simulink model "sampleModel7424_pp_1_1"  (R2018a)
settings: Solver=VariableStepAuto  StartTime=0.0  StopTime=10.0  RelTol=1e-3
undefined symbols (not defined in the file): DiscIntNeverNeededParam
libraries: simulink x211
(part 7 of 7)

== matlab function sampleModel7424_pp_1_1/emi_267 ==
  data: o input; e input
function  fcn(o, e)
o_inv = o^-1;
e_inv = e^-1;

emsg = 'sampleModel7424_pp_1_1/emi_267';
 
if(o == e)
    assert(o_inv == e_inv, [emsg ' ; o_inv~=e_inv']);
    return;
end
 
if(o_inv > 0)
    assert(e_inv < 0, [emsg ' ; e_inv>=0']);
else
    assert(e_inv > 0, [emsg ' ; e_inv<=0']);
end

== matlab function sampleModel7424_pp_1_1/cfblk148/cfblk19/emi_269 ==
  data: o input; e input
function  fcn(o, e)
o_inv = o^-1;
e_inv = e^-1;

emsg = 'sampleModel7424_pp_1_1/cfblk148/cfblk19/emi_269';
 
if(o == e)
    assert(o_inv == e_inv, [emsg ' ; o_inv~=e_inv']);
    return;
end
 
if(o_inv > 0)
    assert(e_inv < 0, [emsg ' ; e_inv>=0']);
else
    assert(e_inv > 0, [emsg ' ; e_inv<=0']);
end

== matlab function sampleModel7424_pp_1_1/cfblk140/emi_271 ==
  data: o input; e input
function  fcn(o, e)
o_inv = o^-1;
e_inv = e^-1;

emsg = 'sampleModel7424_pp_1_1/cfblk140/emi_271';
 
if(o == e)
    assert(o_inv == e_inv, [emsg ' ; o_inv~=e_inv']);
    return;
end
 
if(o_inv > 0)
    assert(e_inv < 0, [emsg ' ; e_inv>=0']);
else
    assert(e_inv > 0, [emsg ' ; e_inv<=0']);
end

== matlab function sampleModel7424_pp_1_1/emi_273 ==
  data: o input; e input
function  fcn(o, e)
o_inv = o^-1;
e_inv = e^-1;

emsg = 'sampleModel7424_pp_1_1/emi_273';
 
if(o == e)
    assert(o_inv == e_inv, [emsg ' ; o_inv~=e_inv']);
    return;
end
 
if(o_inv > 0)
    assert(e_inv < 0, [emsg ' ; e_inv>=0']);
else
    assert(e_inv > 0, [emsg ' ; e_inv<=0']);
end

== matlab function sampleModel7424_pp_1_1/cfblk124/emi_275 ==
  data: o input; e input
function  fcn(o, e)
o_inv = o^-1;
e_inv = e^-1;

emsg = 'sampleModel7424_pp_1_1/cfblk124/emi_275';
 
if(o == e)
    assert(o_inv == e_inv, [emsg ' ; o_inv~=e_inv']);
    return;
end
 
if(o_inv > 0)
    assert(e_inv < 0, [emsg ' ; e_inv>=0']);
else
    assert(e_inv > 0, [emsg ' ; e_inv<=0']);
end

== matlab function sampleModel7424_pp_1_1/cfblk134/cfblk19/emi_277 ==
  data: o input; e input
function  fcn(o, e)
o_inv = o^-1;
e_inv = e^-1;

emsg = 'sampleModel7424_pp_1_1/cfblk134/cfblk19/emi_277';
 
if(o == e)
    assert(o_inv == e_inv, [emsg ' ; o_inv~=e_inv']);
    return;
end
 
if(o_inv > 0)
    assert(e_inv < 0, [emsg ' ; e_inv>=0']);
else
    assert(e_inv > 0, [emsg ' ; e_inv<=0']);
end

== matlab function sampleModel7424_pp_1_1/cfblk125/emi_279 ==
  data: o input; e input
function  fcn(o, e)
o_inv = o^-1;
e_inv = e^-1;

emsg = 'sampleModel7424_pp_1_1/cfblk125/emi_279';
 
if(o == e)
    assert(o_inv == e_inv, [emsg ' ; o_inv~=e_inv']);
    return;
end
 
if(o_inv > 0)
    assert(e_inv < 0, [emsg ' ; e_inv>=0']);
else
    assert(e_inv > 0, [emsg ' ; e_inv<=0']);
end

== matlab function sampleModel7424_pp_1_1/cfblk125/cfblk12/emi_281 ==
  data: o input; e input
function  fcn(o, e)
o_inv = o^-1;
e_inv = e^-1;

emsg = 'sampleModel7424_pp_1_1/cfblk125/cfblk12/emi_281';
 
if(o == e)
    assert(o_inv == e_inv, [emsg ' ; o_inv~=e_inv']);
    return;
end
 
if(o_inv > 0)
    assert(e_inv < 0, [emsg ' ; e_inv>=0']);
else
    assert(e_inv > 0, [emsg ' ; e_inv<=0']);
end

== matlab function sampleModel7424_pp_1_1/cfblk134/cfblk19/emi_283 ==
  data: o input; e input
function  fcn(o, e)
o_inv = o^-1;
e_inv = e^-1;

emsg = 'sampleModel7424_pp_1_1/cfblk134/cfblk19/emi_283';
 
if(o == e)
    assert(o_inv == e_inv, [emsg ' ; o_inv~=e_inv']);
    return;
end
 
if(o_inv > 0)
    assert(e_inv < 0, [emsg ' ; e_inv>=0']);
else
    assert(e_inv > 0, [emsg ' ; e_inv<=0']);
end

== matlab function sampleModel7424_pp_1_1/cfblk134/emi_285 ==
  data: o input; e input
function  fcn(o, e)
o_inv = o^-1;
e_inv = e^-1;

emsg = 'sampleModel7424_pp_1_1/cfblk134/emi_285';
 
if(o == e)
    assert(o_inv == e_inv, [emsg ' ; o_inv~=e_inv']);
    return;
end
 
if(o_inv > 0)
    assert(e_inv < 0, [emsg ' ; e_inv>=0']);
else
    assert(e_inv > 0, [emsg ' ; e_inv<=0']);
end

== matlab function sampleModel7424_pp_1_1/cfblk126/cfblk15/emi_287 ==
  data: o input; e input
function  fcn(o, e)
o_inv = o^-1;
e_inv = e^-1;

emsg = 'sampleModel7424_pp_1_1/cfblk126/cfblk15/emi_287';
 
if(o == e)
    assert(o_inv == e_inv, [emsg ' ; o_inv~=e_inv']);
    return;
end
 
if(o_inv > 0)
    assert(e_inv < 0, [emsg ' ; e_inv>=0']);
else
    assert(e_inv > 0, [emsg ' ; e_inv<=0']);
end

== matlab function sampleModel7424_pp_1_1/cfblk125/cfblk12/emi_289 ==
  data: o input; e input
function  fcn(o, e)
o_inv = o^-1;
e_inv = e^-1;

emsg = 'sampleModel7424_pp_1_1/cfblk125/cfblk12/emi_289';
 
if(o == e)
    assert(o_inv == e_inv, [emsg ' ; o_inv~=e_inv']);
    return;
end
 
if(o_inv > 0)
    assert(e_inv < 0, [emsg ' ; e_inv>=0']);
else
    assert(e_inv > 0, [emsg ' ; e_inv<=0']);
end

== matlab function sampleModel7424_pp_1_1/cfblk127/emi_291 ==
  data: o input; e input
function  fcn(o, e)
o_inv = o^-1;
e_inv = e^-1;

emsg = 'sampleModel7424_pp_1_1/cfblk127/emi_291';
 
if(o == e)
    assert(o_inv == e_inv, [emsg ' ; o_inv~=e_inv']);
    return;
end
 
if(o_inv > 0)
    assert(e_inv < 0, [emsg ' ; e_inv>=0']);
else
    assert(e_inv > 0, [emsg ' ; e_inv<=0']);
end

== matlab function sampleModel7424_pp_1_1/cfblk126/cfblk13/emi_293 ==
  data: o input; e input
function  fcn(o, e)
o_inv = o^-1;
e_inv = e^-1;

emsg = 'sampleModel7424_pp_1_1/cfblk126/cfblk13/emi_293';
 
if(o == e)
    assert(o_inv == e_inv, [emsg ' ; o_inv~=e_inv']);
    return;
end
 
if(o_inv > 0)
    assert(e_inv < 0, [emsg ' ; e_inv>=0']);
else
    assert(e_inv > 0, [emsg ' ; e_inv<=0']);
end

== matlab function sampleModel7424_pp_1_1/emi_295 ==
  data: o input; e input
function  fcn(o, e)
o_inv = o^-1;
e_inv = e^-1;

emsg = 'sampleModel7424_pp_1_1/emi_295';
 
if(o == e)
    assert(o_inv == e_inv, [emsg ' ; o_inv~=e_inv']);
    return;
end
 
if(o_inv > 0)
    assert(e_inv < 0, [emsg ' ; e_inv>=0']);
else
    assert(e_inv > 0, [emsg ' ; e_inv<=0']);
end

== matlab function sampleModel7424_pp_1_1/cfblk138/emi_297 ==
  data: o input; e input
function  fcn(o, e)
o_inv = o^-1;
e_inv = e^-1;

emsg = 'sampleModel7424_pp_1_1/cfblk138/emi_297';
 
if(o == e)
    assert(o_inv == e_inv, [emsg ' ; o_inv~=e_inv']);
    return;
end
 
if(o_inv > 0)
    assert(e_inv < 0, [emsg ' ; e_inv>=0']);
else
    assert(e_inv > 0, [emsg ' ; e_inv<=0']);
end

== matlab function sampleModel7424_pp_1_1/cfblk134/cfblk19/emi_299 ==
  data: o input; e input
function  fcn(o, e)
o_inv = o^-1;
e_inv = e^-1;

emsg = 'sampleModel7424_pp_1_1/cfblk134/cfblk19/emi_299';
 
if(o == e)
    assert(o_inv == e_inv, [emsg ' ; o_inv~=e_inv']);
    return;
end
 
if(o_inv > 0)
    assert(e_inv < 0, [emsg ' ; e_inv>=0']);
else
    assert(e_inv > 0, [emsg ' ; e_inv<=0']);
end

== matlab function sampleModel7424_pp_1_1/cfblk124/cfblk17/emi_301 ==
  data: o input; e input
function  fcn(o, e)
o_inv = o^-1;
e_inv = e^-1;

emsg = 'sampleModel7424_pp_1_1/cfblk124/cfblk17/emi_301';
 
if(o == e)
    assert(o_inv == e_inv, [emsg ' ; o_inv~=e_inv']);
    return;
end
 
if(o_inv > 0)
    assert(e_inv < 0, [emsg ' ; e_inv>=0']);
else
    assert(e_inv > 0, [emsg ' ; e_inv<=0']);
end

== matlab function sampleModel7424_pp_1_1/emi_303 ==
  data: o input; e input
function  fcn(o, e)
o_inv = o^-1;
e_inv = e^-1;

emsg = 'sampleModel7424_pp_1_1/emi_303';
 
if(o == e)
    assert(o_inv == e_inv, [emsg ' ; o_inv~=e_inv']);
    return;
end
 
if(o_inv > 0)
    assert(e_inv < 0, [emsg ' ; e_inv>=0']);
else
    assert(e_inv > 0, [emsg ' ; e_inv<=0']);
end

== matlab function sampleModel7424_pp_1_1/cfblk140/emi_305 ==
  data: o input; e input
function  fcn(o, e)
o_inv = o^-1;
e_inv = e^-1;

emsg = 'sampleModel7424_pp_1_1/cfblk140/emi_305';
 
if(o == e)
    assert(o_inv == e_inv, [emsg ' ; o_inv~=e_inv']);
    return;
end
 
if(o_inv > 0)
    assert(e_inv < 0, [emsg ' ; e_inv>=0']);
else
    assert(e_inv > 0, [emsg ' ; e_inv<=0']);
end

== matlab function sampleModel7424_pp_1_1/cfblk142/emi_307 ==
  data: o input; e input
function  fcn(o, e)
o_inv = o^-1;
e_inv = e^-1;

emsg = 'sampleModel7424_pp_1_1/cfblk142/emi_307';
 
if(o == e)
    assert(o_inv == e_inv, [emsg ' ; o_inv~=e_inv']);
    return;
end
 
if(o_inv > 0)
    assert(e_inv < 0, [emsg ' ; e_inv>=0']);
else
    assert(e_inv > 0, [emsg ' ; e_inv<=0']);
end

== matlab function sampleModel7424_pp_1_1/cfblk125/emi_309 ==
  data: o input; e input
function  fcn(o, e)
o_inv = o^-1;
e_inv = e^-1;

emsg = 'sampleModel7424_pp_1_1/cfblk125/emi_309';
 
if(o == e)
    assert(o_inv == e_inv, [emsg ' ; o_inv~=e_inv']);
    return;
end
 
if(o_inv > 0)
    assert(e_inv < 0, [emsg ' ; e_inv>=0']);
else
    assert(e_inv > 0, [emsg ' ; e_inv<=0']);
end

== matlab function sampleModel7424_pp_1_1/cfblk136/emi_311 ==
  data: o input; e input
function  fcn(o, e)
o_inv = o^-1;
e_inv = e^-1;

emsg = 'sampleModel7424_pp_1_1/cfblk136/emi_311';
 
if(o == e)
    assert(o_inv == e_inv, [emsg ' ; o_inv~=e_inv']);
    return;
end
 
if(o_inv > 0)
    assert(e_inv < 0, [emsg ' ; e_inv>=0']);
else
    assert(e_inv > 0, [emsg ' ; e_inv<=0']);
end

== matlab function sampleModel7424_pp_1_1/cfblk125/cfblk12/emi_313 ==
  data: o input; e input
function  fcn(o, e)
o_inv = o^-1;
e_inv = e^-1;

emsg = 'sampleModel7424_pp_1_1/cfblk125/cfblk12/emi_313';
 
if(o == e)
    assert(o_inv == e_inv, [emsg ' ; o_inv~=e_inv']);
    return;
end
 
if(o_inv > 0)
    assert(e_inv < 0, [emsg ' ; e_inv>=0']);
else
    assert(e_inv > 0, [emsg ' ; e_inv<=0']);
end

== matlab function sampleModel7424_pp_1_1/cfblk134/emi_315 ==
  data: o input; e input
function  fcn(o, e)
o_inv = o^-1;
e_inv = e^-1;

emsg = 'sampleModel7424_pp_1_1/cfblk134/emi_315';
 
if(o == e)
    assert(o_inv == e_inv, [emsg ' ; o_inv~=e_inv']);
    return;
end
 
if(o_inv > 0)
    assert(e_inv < 0, [emsg ' ; e_inv>=0']);
else
    assert(e_inv > 0, [emsg ' ; e_inv<=0']);
end

== matlab function sampleModel7424_pp_1_1/cfblk134/emi_317 ==
  data: o input; e input
function  fcn(o, e)
o_inv = o^-1;
e_inv = e^-1;

emsg = 'sampleModel7424_pp_1_1/cfblk134/emi_317';
 
if(o == e)
    assert(o_inv == e_inv, [emsg ' ; o_inv~=e_inv']);
    return;
end
 
if(o_inv > 0)
    assert(e_inv < 0, [emsg ' ; e_inv>=0']);
else
    assert(e_inv > 0, [emsg ' ; e_inv<=0']);
end

== matlab function sampleModel7424_pp_1_1/cfblk126/cfblk15/emi_319 ==
  data: o input; e input
function  fcn(o, e)
o_inv = o^-1;
e_inv = e^-1;

emsg = 'sampleModel7424_pp_1_1/cfblk126/cfblk15/emi_319';
 
if(o == e)
    assert(o_inv == e_inv, [emsg ' ; o_inv~=e_inv']);
    return;
end
 
if(o_inv > 0)
    assert(e_inv < 0, [emsg ' ; e_inv>=0']);
else
    assert(e_inv > 0, [emsg ' ; e_inv<=0']);
end

== matlab function sampleModel7424_pp_1_1/cfblk148/cfblk19/emi_321 ==
  data: o input; e input
function  fcn(o, e)
o_inv = o^-1;
e_inv = e^-1;

emsg = 'sampleModel7424_pp_1_1/cfblk148/cfblk19/emi_321';
 
if(o == e)
    assert(o_inv == e_inv, [emsg ' ; o_inv~=e_inv']);
    return;
end
 
if(o_inv > 0)
    assert(e_inv < 0, [emsg ' ; e_inv>=0']);
else
    assert(e_inv > 0, [emsg ' ; e_inv<=0']);
end

== matlab function sampleModel7424_pp_1_1/cfblk124/cfblk17/emi_323 ==
  data: o input; e input
function  fcn(o, e)
o_inv = o^-1;
e_inv = e^-1;

emsg = 'sampleModel7424_pp_1_1/cfblk124/cfblk17/emi_323';
 
if(o == e)
    assert(o_inv == e_inv, [emsg ' ; o_inv~=e_inv']);
    return;
end
 
if(o_inv > 0)
    assert(e_inv < 0, [emsg ' ; e_inv>=0']);
else
    assert(e_inv > 0, [emsg ' ; e_inv<=0']);
end

== matlab function sampleModel7424_pp_1_1/cfblk130/cfblk12/emi_325 ==
  data: o input; e input
function  fcn(o, e)
o_inv = o^-1;
e_inv = e^-1;

emsg = 'sampleModel7424_pp_1_1/cfblk130/cfblk12/emi_325';
 
if(o == e)
    assert(o_inv == e_inv, [emsg ' ; o_inv~=e_inv']);
    return;
end
 
if(o_inv > 0)
    assert(e_inv < 0, [emsg ' ; e_inv>=0']);
else
    assert(e_inv > 0, [emsg ' ; e_inv<=0']);
end

== matlab function sampleModel7424_pp_1_1/cfblk124/cfblk15/emi_327 ==
  data: o input; e input
function  fcn(o, e)
o_inv = o^-1;
e_inv = e^-1;

emsg = 'sampleModel7424_pp_1_1/cfblk124/cfblk15/emi_327';
 
if(o == e)
    assert(o_inv == e_inv, [emsg ' ; o_inv~=e_inv']);
    return;
end
 
if(o_inv > 0)
    assert(e_inv < 0, [emsg ' ; e_inv>=0']);
else
    assert(e_inv > 0, [emsg ' ; e_inv<=0']);
end

== matlab function sampleModel7424_pp_1_1/emi_329 ==
  data: o input; e input
function  fcn(o, e)
o_inv = o^-1;
e_inv = e^-1;

emsg = 'sampleModel7424_pp_1_1/emi_329';
 
if(o == e)
    assert(o_inv == e_inv, [emsg ' ; o_inv~=e_inv']);
    return;
end
 
if(o_inv > 0)
    assert(e_inv < 0, [emsg ' ; e_inv>=0']);
else
    assert(e_inv > 0, [emsg ' ; e_inv<=0']);
end

== matlab function sampleModel7424_pp_1_1/cfblk148/cfblk19/emi_331 ==
  data: o input; e input
function  fcn(o, e)
o_inv = o^-1;
e_inv = e^-1;

emsg = 'sampleModel7424_pp_1_1/cfblk148/cfblk19/emi_331';
 
if(o == e)
    assert(o_inv == e_inv, [emsg ' ; o_inv~=e_inv']);
    return;
end
 
if(o_inv > 0)
    assert(e_inv < 0, [emsg ' ; e_inv>=0']);
else
    assert(e_inv > 0, [emsg ' ; e_inv<=0']);
end

== matlab function sampleModel7424_pp_1_1/cfblk127/emi_333 ==
  data: o input; e input
function  fcn(o, e)
o_inv = o^-1;
e_inv = e^-1;

emsg = 'sampleModel7424_pp_1_1/cfblk127/emi_333';
 
if(o == e)
    assert(o_inv == e_inv, [emsg ' ; o_inv~=e_inv']);
    return;
end
 
if(o_inv > 0)
    assert(e_inv < 0, [emsg ' ; e_inv>=0']);
else
    assert(e_inv > 0, [emsg ' ; e_inv<=0']);
end

== matlab function sampleModel7424_pp_1_1/cfblk148/cfblk19/emi_335 ==
  data: o input; e input
function  fcn(o, e)
o_inv = o^-1;
e_inv = e^-1;

emsg = 'sampleModel7424_pp_1_1/cfblk148/cfblk19/emi_335';
 
if(o == e)
    assert(o_inv == e_inv, [emsg ' ; o_inv~=e_inv']);
    return;
end
 
if(o_inv > 0)
    assert(e_inv < 0, [emsg ' ; e_inv>=0']);
else
    assert(e_inv > 0, [emsg ' ; e_inv<=0']);
end

== matlab function sampleModel7424_pp_1_1/cfblk148/cfblk19/emi_337 ==
  data: o input; e input
function  fcn(o, e)
o_inv = o^-1;
e_inv = e^-1;

emsg = 'sampleModel7424_pp_1_1/cfblk148/cfblk19/emi_337';
 
if(o == e)
    assert(o_inv == e_inv, [emsg ' ; o_inv~=e_inv']);
    return;
end
 
if(o_inv > 0)
    assert(e_inv < 0, [emsg ' ; e_inv>=0']);
else
    assert(e_inv > 0, [emsg ' ; e_inv<=0']);
end

== matlab function sampleModel7424_pp_1_1/cfblk130/emi_339 ==
  data: o input; e input
function  fcn(o, e)
o_inv = o^-1;
e_inv = e^-1;

emsg = 'sampleModel7424_pp_1_1/cfblk130/emi_339';
 
if(o == e)
    assert(o_inv == e_inv, [emsg ' ; o_inv~=e_inv']);
    return;
end
 
if(o_inv > 0)
    assert(e_inv < 0, [emsg ' ; e_inv>=0']);
else
    assert(e_inv > 0, [emsg ' ; e_inv<=0']);
end

== matlab function sampleModel7424_pp_1_1/cfblk124/emi_341 ==
  data: o input; e input
function  fcn(o, e)
o_inv = o^-1;
e_inv = e^-1;

emsg = 'sampleModel7424_pp_1_1/cfblk124/emi_341';
 
if(o == e)
    assert(o_inv == e_inv, [emsg ' ; o_inv~=e_inv']);
    return;
end
 
if(o_inv > 0)
    assert(e_inv < 0, [emsg ' ; e_inv>=0']);
else
    assert(e_inv > 0, [emsg ' ; e_inv<=0']);
end
